simulink model "model_zad2"  (Simulink 8.1)
settings: Solver=ode45  StartTime=0.0  StopTime=Tsim  RelTol=1e-3
values from neighbouring files (symbols this model uses):
  c = 1    [inicijalizacija.m]    (also in model_sfun.m)
  k = 100    [inicijalizacija.m]    (also in model_sfun.m)
  m = 3    [inicijalizacija.m]    (also in model_sfun.m = 2)
  Ts = dt    [inicijalizacija.m]
libraries: simulink x2
settings Model: Creator=mladen  LastModifiedBy=Nikola
settings DataIOCC: SignalLoggingSaveFormat=Dataset
settings OptimizationCC: ExpressionDepthLimit=128
settings DebuggingCC: FcnCallInpInsideContextMsg=EnableAllAsError  StateNameClashWarn=none
settings GRTTargetCC: CodeReplacementLibrary=C89/C90 (ANSI)  CombineOutputUpdateFcns=on  GRTInterface=off

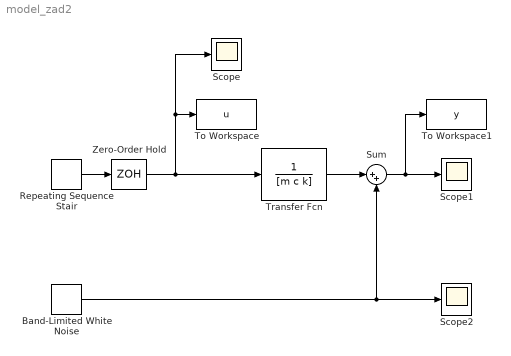
== system model_zad2 ==
  Band-Limited White Noise : simulink/Sources/Band-Limited White Noise  Cov=[0.000001]  Ts=Ts  seed=randi(23341,1,1)
  Repeating Sequence Stair : simulink/Sources/Repeating Sequence Stair  OutValues=Ui  tsamp=Ts  OutMin=[]  OutMax=[]  OutDataTypeStr=double  OutputDataTypeScalingMode=double  OutDataType=fixdt(0,8)  ConRadixGroup=Best Precision: Vector-wise  OutScaling=2^-12
  Scope : Scope
  Scope1 : Scope
      settings: SampleInput=on  SampleTime=0.001
  Scope2 : Scope
      settings: SaveName=ScopeData2
  Sum : Sum  Inputs=|++
  To Workspace : ToWorkspace  VariableName=u  SaveFormat=Structure With Time  SampleTime=Ts
  To Workspace1 : ToWorkspace  VariableName=y  SaveFormat=Structure With Time  SampleTime=Ts
  Transfer Fcn : TransferFcn  Denominator=[m c k]
  Zero-Order Hold : ZeroOrderHold  SampleTime=Ts
  wires:
  Transfer Fcn/1 -> Sum/1
  Sum/1 -> To Workspace1/1, Scope1/1
  Repeating Sequence Stair/1 -> Zero-Order Hold/1
  Zero-Order Hold/1 -> Transfer Fcn/1, To Workspace/1, Scope/1
  Band-Limited White Noise/1 -> Sum/2, Scope2/1
